simulink model "lab3_2"  (R2014b)
settings: Solver=ode45  StartTime=0.0  StopTime=5  RelTol=1e-3
settings Model: Creator=StudentPA  LastModifiedBy=StudentPA

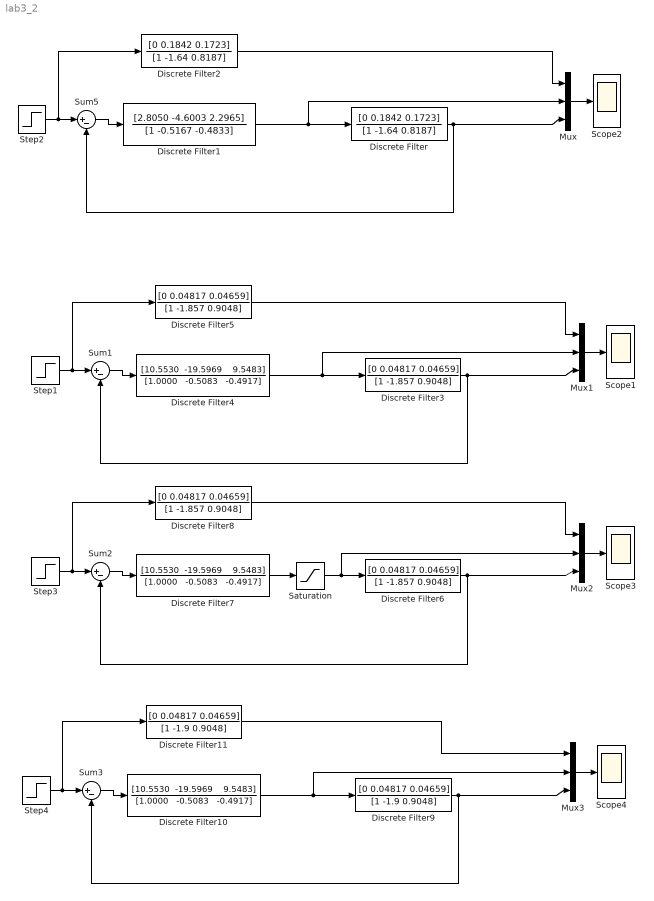
== system lab3_2 ==
  Discrete Filter : DiscreteFilter  Numerator=[0 0.1842 0.1723]  Denominator=[1 -1.64 0.8187]  SampleTime=0.1
  Discrete Filter1 : DiscreteFilter  Numerator=[2.8050 -4.6003 2.2965]  Denominator=[1 -0.5167 -0.4833]  SampleTime=0.1
  Discrete Filter10 : DiscreteFilter  Numerator="[10.5530  -19.5969    9.5483]"  Denominator="[1.0000   -0.5083   -0.4917]"  SampleTime=0.05
  Discrete Filter11 : DiscreteFilter  Numerator=[0 0.04817 0.04659]  Denominator=[1 -1.9 0.9048]  SampleTime=0.05
  Discrete Filter2 : DiscreteFilter  Numerator=[0 0.1842 0.1723]  Denominator=[1 -1.64 0.8187]  SampleTime=0.1
  Discrete Filter{3,5..6,8} (4 alike) : DiscreteFilter  Numerator=[0 0.04817 0.04659]  Denominator=[1 -1.857 0.9048]  SampleTime=0.05
  Discrete Filter4 : DiscreteFilter  Numerator="[10.5530  -19.5969    9.5483]"  Denominator="[1.0000   -0.5083   -0.4917]"  SampleTime=0.05
  Discrete Filter7 : DiscreteFilter  Numerator="[10.5530  -19.5969    9.5483]"  Denominator="[1.0000   -0.5083   -0.4917]"  SampleTime=0.05
  Discrete Filter9 : DiscreteFilter  Numerator=[0 0.04817 0.04659]  Denominator=[1 -1.9 0.9048]  SampleTime=0.05
  Mux{,1..3} (4 alike) : Mux  Inputs=3
  Saturation : Saturate  UpperLimit=3  LowerLimit=-3  SampleTime=0.05
  Scope{1..4} (4 alike) : Scope
      Scope1 settings: ShowLegends=on  YMin=0  YMax=2
      Scope2 settings: ShowLegends=on  YMin=0  YMax=2  SaveName=ScopeData2
      Scope3 settings: ShowLegends=on  YMin=0  YMax=2
      Scope4 settings: ShowLegends=on  YMin=0  YMax=2  SaveName=ScopeData3
  Step1 : Step  Time=0  SampleTime=0.05
  Step2 : Step  Time=0  SampleTime=0.1
  Step3 : Step  Time=0  SampleTime=0.05
  Step4 : Step  Time=0  SampleTime=0.05
  Sum{1..3,5} (4 alike) : Sum  Inputs=|+-
  wires:
  Step2/1 -> Discrete Filter2/1, Sum5/1
  Discrete Filter1/1 -> Mux/2, Discrete Filter/1
  Sum5/1 -> Discrete Filter1/1
  Discrete Filter/1 -> Mux/3, Sum5/2
  Discrete Filter2/1 -> Mux/1
  Mux/1 -> Scope2/1
  Step1/1 -> Sum1/1, Discrete Filter5/1
  Discrete Filter4/1 -> Discrete Filter3/1, Mux1/2
  Sum1/1 -> Discrete Filter4/1
  Discrete Filter3/1 -> Sum1/2, Mux1/3
  Discrete Filter5/1 -> Mux1/1
  Mux1/1 -> Scope1/1
  Step3/1 -> Discrete Filter8/1, Sum2/1
  Sum2/1 -> Discrete Filter7/1
  Discrete Filter6/1 -> Mux2/3, Sum2/2
  Discrete Filter8/1 -> Mux2/1
  Mux2/1 -> Scope3/1
  Saturation/1 -> Mux2/2, Discrete Filter6/1
  Discrete Filter7/1 -> Saturation/1
  Step4/1 -> Discrete Filter11/1, Sum3/1
  Discrete Filter10/1 -> Mux3/2, Discrete Filter9/1
  Sum3/1 -> Discrete Filter10/1
  Discrete Filter9/1 -> Mux3/3, Sum3/2
  Mux3/1 -> Scope4/1
  Discrete Filter11/1 -> Mux3/1
